simulink model "manip_levitation"  (Simulink 7.2)
settings: Solver=ode1  SolverMode=SingleTasking  StartTime=0.0  StopTime=Inf  FixedStep=1/1000  RelTol=1e-3
PostLoadFcn:
  | , if any(exist('dsrtsu_mdlpostloadfcn', 'file') == [2, 3, 6]), try dsrtsu_mdlpostloadfcn('Execute', bdroot); catch fprintf('Error in PostLoadFcn (dsrtsu_mdlpostloadfcn) for model "%s":\n %s\n', bdroot, lasterr); end, end,
libraries: rti4201serlib x3, rtilibm x1
settings Model: DSRTSU_INTERNAL_RTI_VER=330  DSRTSU_INTERNAL_RTI_TYPE=rti1005  Creator=stephane.oster  LastModifiedBy=joel.abadie  ExtModeTrigMode=oneshot  ExtModeArmWhenConnect=off  BufferReuse=off
settings OptimizationCC: BlockReduction=off  ConditionallyExecuteInputs=off  InlineInvariantSignals=on  OptimizeBlockIOStorage=off  BufferReuse=off  ExpressionFolding=off  LocalBlockOutputs=off  InitFltsAndDblsToZero=on
settings DebuggingCC: SaveWithParameterizedLinksMsg=none  SignalResolutionControl=TryResolveAllWithWarning  MultiTaskDSMMsg=warning  MultiTaskCondExecSysMsg=none  MultiTaskRateTransMsg=warning  TasksWithSamePriorityMsg=none  StrictBusMsg=None
settings HardwareCC: ProdIntDivRoundTo=Zero  ProdEndianess=BigEndian  ProdHWDeviceType=Specified  TargetIntDivRoundTo=Zero  TargetEndianess=BigEndian
settings RTWCC: SystemTargetFile=rti1005.tlc  MakeCommand=make_rti  TemplateMakefile=rti1005.tmf  Description=dSPACE DS1005 Hardware Platform  RTWVerbose=off  ProcessScript=rti1005_make_rtw_hook  CustomInclude=g:\bin_jabadie  IncludeERTFirstTime=on
settings STFCustomTargetCC: SystemTargetFile=rti1005.tlc
settings GRTTargetCC: CompOptLevelCompliant=off  MatFileLogging=off  ExtModeMexFile=noextcomm
settings CustomProperty: DataType=RTWOptions_EnumType_C__dSPACE_matlab_rti1005_tlc_rti1005_InitialSimState  Value=RUN
settings EnumStrPairs: String=RUN

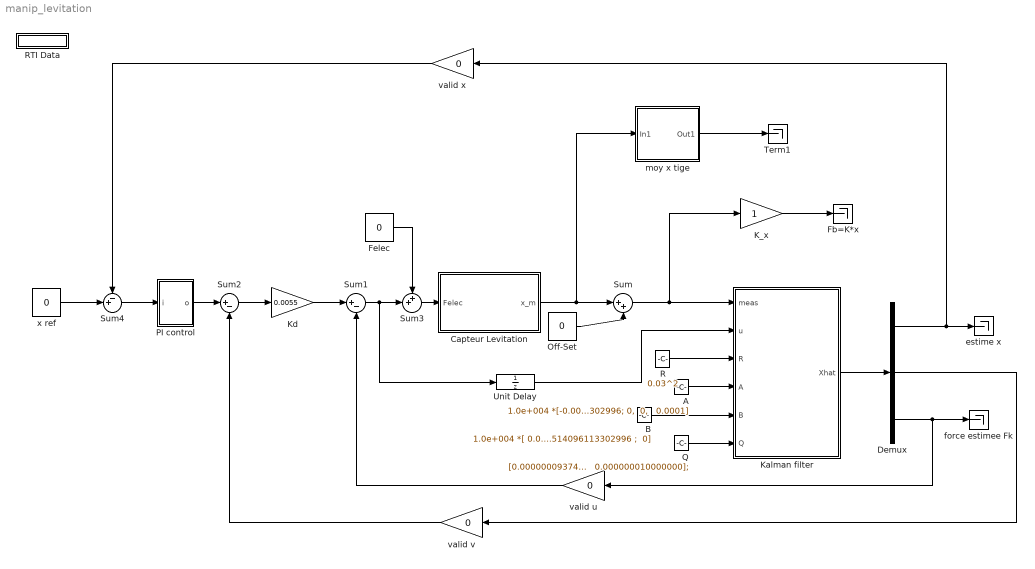
== system manip_levitation ==
  A : Constant  Value="1.0e+004 *[-0.000041693801048, 0.000000021197346, 0.000610749142449; -0.351270298286295, -0.000044721993275, 1.514096113302996; 0,  0,   0.0001]"
  B : Constant  Value=|
      | 1.0e+004 *[ 0.000610749142449;
      |    1.514096113302996;
      |  0]
  Capteur Levitation : Subsystem
  Demux : Demux  Outputs=3
  Fb=K*x : Terminator
  Felec : Constant  Value=0  OutDataType=sfix(16)  OutScaling=2^0
  K_x : Gain  ParameterDataType=sfix(16)  ParameterScaling=2^0  OutDataType=sfix(16)  OutScaling=2^0
  Kalman filter : Stateflow chart  TreatAsAtomicUnit=on
  Kd : Gain  Gain=0.0055  ParameterDataType=sfix(16)  ParameterScaling=2^0  OutDataType=sfix(16)  OutScaling=2^0
  Off-Set : Constant  Value=0  OutDataType=sfix(16)  OutScaling=2^0
  PI control : Subsystem
  Q : Constant  Value=|
      | [0.000000093740541   0.000373014515003   0.000000023776859;
      |    0.000373014515003   1.757821222396016   0.000122149828490;
      |    0.000000023776859,   0.000122149828490,   0.000000010000000];
  R : Constant  Value=0.03^2
  RTI Data : Subsystem  Tag=struct('RTIDataServer',struct('RTIModelDescription','struct(''main'',''manip_levitation'',''sub'','''',''isMp'',0)'))  LoadFcn="if exist('rtidc'), try,  rtidc('DataHostBlockClbLoad', gcbh); catch, disp(['Warning: ''LoadFcn'' for RTI Data block failed: ' lasterr]); end, end,"
      settings: CopyFcn="if exist('rtidc'), try,  rtidc('DataHostBlockClbCopy', gcbh); catch, disp(['Warning: ''CopyFcn'' for RTI Data block failed: ' lasterr]); end, end,"  DeleteFcn="if exist('rtidc'), try,  rtidc('DataHostBlockClbDelete', gcbh); catch, disp(['Warning: ''DeleteFcn'' for RTI Data block failed: ' lasterr]); end, end,"  ModelCloseFcn="if exist('rtidc'), try,  rtidc('DataHostBlockClbModelClose', gcbh); catch, disp(['Warning: ''ModelCloseFcn'' for RTI Data block failed: ' lasterr]); end, end,"  PreSaveFcn="if exist('rtidc'), try,  rtidc('DataHostBlockClbPreSave', gcbh); catch, disp(['Warning: ''PreSaveFcn'' for RTI Data block failed: ' lasterr]); end, end,"  PostSaveFcn="if exist('rtidc'), try,  rtidc('DataHostBlockClbPostSave', gcbh); catch, disp(['Warning: ''PostSaveFcn'' for RTI Data block failed: ' lasterr]); end, end,"  NameChangeFcn="if exist('rtidc'), try,  rtidc('DataHostBlockClbNameChange', gcbh); catch, disp(['Warning: ''NameChangeFcn'' for RTI Data block failed: ' lasterr]); end, end,"
      mask Type: RTI_DATA_HOST
      mask Description:
      | RTI Data Block.
      | This block is used by RTI to store internal model-dependent data.
      | Please keep this block on the root level of the model. Deleting this block will result in data loss.
      | 
      | NEVER DELETE OR COPY THIS BLOCK!
      mask Help:
      | RTI Data Block.
      | This block is used by RTI to store internal model-dependent data.
      | Please keep this block on the root level of the model. Deleting this block will result in data loss.
      | 
      | NEVER DELETE OR COPY THIS BLOCK!
      mask Display:
      | text(0.5, 0.5, 'RTI Data', 'HorizontalAlignment', 'center');
      | plot([1 0]);
  Sum : Sum  Inputs=|++  OutDataType=sfix(16)  OutScaling=2^0
  Sum1 : Sum  Inputs=|+-  OutDataType=sfix(16)  OutScaling=2^0
  Sum2 : Sum  Inputs=|+-  OutDataType=sfix(16)  OutScaling=2^0
  Sum3 : Sum  Inputs=++|  OutDataType=sfix(16)  OutScaling=2^0
  Sum4 : Sum  Inputs=-+|  OutDataType=sfix(16)  OutScaling=2^0
  Term1 : Terminator
  Unit Delay : UnitDelay  SampleTime=-1
  estime x : Terminator
  force estimee Fk : Terminator
  moy x tige : Subsystem  mask(s fonction jabadie){duree=2, T_m=0.01, to=2}
      mask prompts: duree "duree du moyennage (s)"; T_m "periode d echatillonage moyennage (s)"; to "constante de temp du filtre (s)"
      mask help:
      | sort une valeur moyenne d'un signal
      | sur une duree donnee puis applique un filtre
      | du premier ordre
  valid u : Gain  Orientation=left  Gain=0  ParameterDataType=sfix(16)  ParameterScaling=2^0  OutDataType=sfix(16)  OutScaling=2^0
  valid v : Gain  Orientation=left  Gain=0  ParameterDataType=sfix(16)  ParameterScaling=2^0  OutDataType=sfix(16)  OutScaling=2^0
  valid x : Gain  Orientation=left  Gain=0  ParameterDataType=sfix(16)  ParameterScaling=2^0  OutDataType=sfix(16)  OutScaling=2^0
  x ref : Constant  Value=0  OutDataType=sfix(16)  OutScaling=2^0
  wires:
  Demux/1 -> estime x/1, valid x/1
  Demux/3 -> force estimee Fk/1, valid u/1
  Sum/1 -> K_x/1, Kalman filter/1(meas)
  Off-Set/1 -> Sum/2
  moy x tige/1(Out1) -> Term1/1
  K_x/1 -> Fb=K*x/1
  Capteur Levitation/1(x_m) -> Sum/1, moy x tige/1(In1)
  Sum1/1 -> Unit Delay/1, Sum3/2
  Kalman filter/1(Xhat) -> Demux/1
  Demux/2 -> valid v/1
  R/1 -> Kalman filter/3(R)
  B/1 -> Kalman filter/5(B)
  A/1 -> Kalman filter/4(A)
  Q/1 -> Kalman filter/6(Q)
  Unit Delay/1 -> Kalman filter/2(u)
  Felec/1 -> Sum3/1
  Sum3/1 -> Capteur Levitation/1(Felec)
  PI control/1(o) -> Sum2/1
  Sum2/1 -> Kd/1
  Kd/1 -> Sum1/1
  valid u/1 -> Sum1/2
  Sum4/1 -> PI control/1(i)
  x ref/1 -> Sum4/2
  valid v/1 -> Sum2/2
  valid x/1 -> Sum4/1

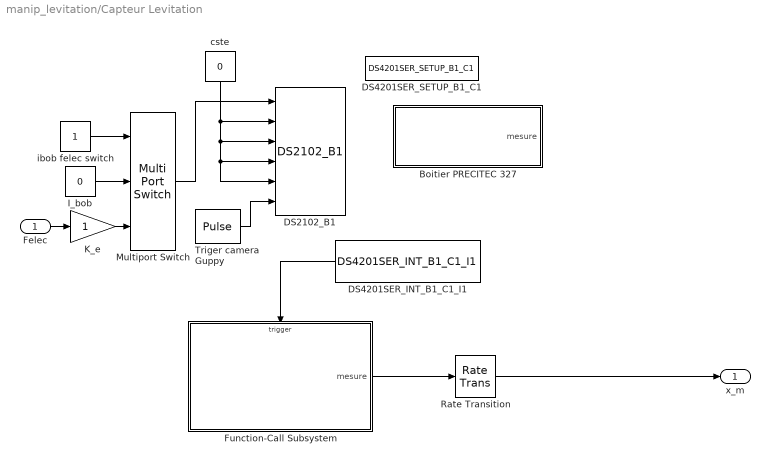
== system manip_levitation/Capteur Levitation ==
  Felec : Inport
  Boitier PRECITEC 327 : Subsystem
  DS2102_B1 : rtilibm/DS2102/DS2102_B1  SystemSampleTime=-1  BoardNo=1  Range=[10 10 10 10 10 0]  IOErrorMode=[1 1 1 1 1 1]  DeglitcherMode=[0 0 0 0 0 0]  InitValue=[0 0 0 0 0 0]  TermMode=[1 1 1 1 1 1]  TermValue=[0 0 0 0 0 0]  DialogFcn=gui2102  UnitName={'DS2102_B'}  UnitValues={ 1 }  DSProperties=struct('RTI',struct('Version',uint32(1),'BlockType',struct('isSLSource',uint8(0),'isSLSink',uint8(1),'isHWSource',uint8(0),'isHWSink',uint8(1),'isSetup',uint8(0),'isInline',uint8(1),'isNonInline',uint8(0),'isInterrupt',uint8(0),'isChannelwise',uint8(0)),'IOBoardType','DS2102','UnitType','DAC','Identifier','DAC','DialogType','ML','BlockSet','NONE','SlaveProcessor','NONE'))
  DS4201SER_INT_B1_C1_I1 : rti4201serlib/DS4201SER_INT_B1_C1_I1  Orientation=left  SystemSampleTime=-1  Reserved1=[]  Reserved2=[]  Reserved3=[]  Reserved4=[]  DSProperties=struct('RTI',struct('IOBoardType',{{'DS4201','SER'}},'SlaveProcessor','NONE','Version',uint32(3),'BlockType',struct('isSLSource',uint8(1),'isSLSink',uint8(0),'isHWSource',uint8(0),'isHWSink',uint8(0),'isSetup',uint8(0),'isInline',uint8(1),'isNonInline',uint8(0),'isInterrupt',uint8(1),'isChannelwise',uint8(1)),'UnitType','GENSER','Identifier','SERINT','DialogType','ML','BlockSet','NONE','RelationId',struct('TH',struct('BlockId','HWINT'))))  RTIBlockInterface=struct('BlockDisplay',{{['DS4201 SER Interrupt\n Board 1 Channel 1\nReceive Interrupt'],'center'}},'BlockName',struct('Token',{{'DS4201SER_INT_B','_C','_I'}},'BlockParam',{{'BoardNo','ChannelNo','IntType'}}),'OutputPortsWidth',int32(1),'OutputPortsActive',1,'OutputPortsName',{{[' ']}},'IconTransparency','off','ParameterTunableNames',{{}},'InitLevel',3,'DialogFcn','guigenserserint','MaskDescription',['To make the interrupts of the UART serial interface available as trigger source.'],'FunctionCall',uint32(0),'Options',{{'SS_OPTION_FORCE_NONINLINED_FCNCALL','SS_OPTION_ASYNCHRONOUS_INTERRUPT'}})  RTIBlockParameters=struct('Class',{{'UART','OFF',[]}},'ClassType',{{1,'OFF',[]}},'BoardType',{{'UART','OFF',[]}},'ThIntNo',{{1,'OFF',[1 4]}},'ThSubIntNo',{{0,'ON',[0 4]}},'ThSrcSgnName',{{['UART RX SW FIFO interrupt'],'OFF',[]}},'IntMode',{{0,'OFF',[]}},'TLCFileName',{{'rti_hwinterrupt','OFF',[]}},'PHSBoardBaseId',{{'DS4201S','OFF',[]}},'BoardNo',{{1,'ON',[1 16]}},'ChannelNo',{{1,'ON',[1 4]}},'ChannelNumOf',{{4,'OFF',[]}},'ThBlk',{{['struct(''blkh'',12.0009765625,''srcId'',''4201SB1I0S0'',''srcSgnId'',''4201SB1I0S0'',''intervalTmrBlockId'',[],''srcSgnName'',[''DS4201S_B1 UART RX SW FIFO interrupt''],''srcCpuId'','''',''isSrcCpu'',1,''isTargetCpu'',1,''srcOnMasterCpu'',1,''boardType'',''DS4201S'',''boardTypeNo'',''4201S'',''boardNo'',1,''intNo'',0,''subIntNo'',0,''period'',0,''entryPoint'',''rti_taskFcn001'',''blockName'',''DS4201SER_INT_B1_C1_I1'',''taskNameDisplayExt'','''',''taskType'',''HWINT'',''groupId'',''SERINT'',''hookFcn'',''NULL'',''isTimerTaskSrc'',0,''service'','''',''mpBlkId'','''',''taskPriorityPreConfig'',''none'',''taskPriority'',-1,''taskSortWeighting'',[],''taskSchedulingPolicy'',''FCFS'',''taskOvrPreConfig'',''none'',''taskOvrStrategy'',1,''taskOvrQueueSize'',1,''taskVisibility'',''on'',''taskGroupId'','''',''taskGroupDisplayOrder'',[],''serviceDynamicGen'',0,''disableCodeGen'',0)'],'OFF',[]}},'IntType',{{1,'ON',[1 4]}},'ReceiveIntLevelFifo',{{'4','OFF',[]}},'IntTypeMacro',{{'DSSER_TRIGGER_LEVEL_SUBINT_MASK','OFF',[]}},'FifoSizeDefault',{{64,'OFF',[]}})  RTISFcnParameters=struct('BoardNo','double','ChannelNo','double','ThIntNo','double','ThSubIntNo','double','ThBlk','struct','IntType','double','ReceiveIntLevelFifo','double','TLCFileName','char','IntTypeMacro','char')  RTIBlockParaDefault=struct('Class','UART','ClassType',1,'BoardType','UART','ThIntNo',1,'ThSubIntNo',0,'ThSrcSgnName',['RX SW FIFO interrupt'],'IntMode',0,'TLCFileName','rti_hwinterrupt','PHSBoardBaseId','DS4201S','BoardNo',1,'ChannelNo',1,'ChannelNumOf',4,'ThBlk',['struct(''srcSgnId'', '''')'],'IntType',1,'ReceiveIntLevelFifo',1,'IntTypeMacro','DSSER_TRIGGER_LEVEL_SUBINT_MASK','FifoSizeDefault',64)
  DS4201SER_SETUP_B1_C1 : rti4201serlib/DS4201SER_SETUP_B1_C1  SystemSampleTime=-1  Reserved1=[]  Reserved2=[]  Reserved3=[]  Reserved4=[]  DSProperties=struct('RTI',struct('Version',uint32(2),'IOBoardType',{{'DS4201','SER'}},'SlaveProcessor','NONE','BlockType',struct('isSLSource',uint8(0),'isSLSink',uint8(0),'isHWSource',uint8(0),'isHWSink',uint8(0),'isSetup',uint8(1),'isInline',uint8(1),'isNonInline',uint8(0),'isInterrupt',uint8(0),'isChannelwise',uint8(1)),'UnitType','GENSER','Identifier','SETUP','DialogType','ML','BlockSet','NONE'))  RTIBlockInterface=struct('BlockName',struct('Token',{{'DS4201SER_SETUP_B','_C'}},'BlockParam',{{'BoardNo','ChannelNo'}}),'BlockDisplay',{{['Serial Setup'],'center'}},'IconTransparency','off','ParameterTunableNames',{{}},'InitLevel',1,'DialogFcn','guigensersetup','MaskDescription',['To set the global specifications for the UART interface.'])  RTIBlockParameters=struct('ParityMode',{{1,'OFF',[1 3]}},'TransceiverMode',{{[1;1;1;1],'OFF',[]}},'QuartzFrequency',{{'1843200','OFF',[]}},'BoardNo',{{1,'ON',[1 16]}},'ChannelNo',{{1,'ON',[1 4]}},'ChannelNumOf',{{4,'OFF',[]}},'BaudRate',{{'115200','OFF',[]}},'DataBitsNumOf',{{4,'OFF',[1 4]}},'StopBitsNumOf',{{1,'OFF',[1 3]}},'ReceiveIntLevelUart',{{2,'OFF',[1 4]}},'AutoflowMode',{{0,'OFF',[]}},'FifoSize',{{'256','OFF',[]}},'ReceiveIntLevelFifo',{{0,'OFF',[]}},'FifoOverrunMode',{{2,'OFF',[]}},'FifoBlockSize',{{'4','OFF',[]}},'TermMode',{{1,'OFF',[]}},'TLCFileName',{{'rtigensersetup','OFF',[]}})  RTISFcnParameters=struct('BoardNo','double','ChannelNo','double','ChannelNumOf','double','BaudRate','double','DataBitsNumOf','double','StopBitsNumOf','double','ParityMode','double','TransceiverMode','double','ReceiveIntLevelUart','double','AutoflowMode','double','FifoSize','double','ReceiveIntLevelFifo','double','FifoBlockSize','double','TermMode','double','QuartzFrequency','double','TLCFileName','char')  RTIBlockParaDefault=struct('ParityMode',1,'TransceiverMode',[1;1;1;1],'QuartzFrequency',1843200,'BoardNo',1,'ChannelNo',1,'ChannelNumOf',4,'BaudRate',115200,'DataBitsNumOf',4,'StopBitsNumOf',1,'ReceiveIntLevelUart',4,'AutoflowMode',0,'FifoSize',64,'ReceiveIntLevelFifo',0,'FifoOverrunMode',1,'FifoBlockSize',0,'TermMode',1,'TLCFileName','rtigensersetup')
  Function-Call Subsystem : Subsystem  TreatAsAtomicUnit=on
  I_bob : Constant  Value=0  OutDataType=sfix(16)  OutScaling=2^0
  K_e : Gain  ParameterDataType=sfix(16)  ParameterScaling=2^0  OutDataType=sfix(16)  OutScaling=2^0
  Multiport Switch : MultiPortSwitch  Inputs=2  OutDataType=sfix(16)  OutScaling=2^0
  Rate Transition : RateTransition  Deterministic=off  OutPortSampleTimeOpt=Inherit
  Triger camera Guppy : DiscretePulseGenerator  PulseType=Time based  Amplitude=0.5  Period=1  PulseWidth=50
  cste : Constant  Orientation=down  Value=0  OutDataType=sfix(16)  OutScaling=2^0
  ibob felec switch : Constant  OutDataType=sfix(16)  OutScaling=2^0
  x_m : Outport
  wires:
  cste/1 -> DS2102_B1/2, DS2102_B1/3, DS2102_B1/4, DS2102_B1/5
  Felec/1 -> K_e/1
  ibob felec switch/1 -> Multiport Switch/1
  K_e/1 -> Multiport Switch/3
  I_bob/1 -> Multiport Switch/2
  DS4201SER_INT_B1_C1_I1/1 -> Function-Call Subsystem/Trigger
  Function-Call Subsystem/1(mesure) -> Rate Transition/1
  Rate Transition/1 -> x_m/1
  Multiport Switch/1 -> DS2102_B1/1
  Triger camera Guppy/1 -> DS2102_B1/6

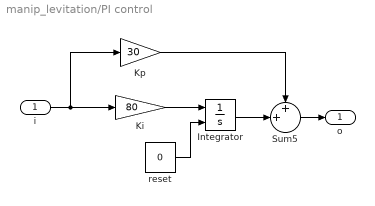
== system manip_levitation/PI control ==
  i : Inport
  Integrator : Integrator  ExternalReset=level
  Ki : Gain  Gain=80  ParameterDataType=sfix(16)  ParameterScaling=2^0  OutDataType=sfix(16)  OutScaling=2^0  SaturateOnIntegerOverflow=on  OutDataTypeStr=Inherit: Same as input  ParamDataTypeStr=Inherit: Same as input
  Kp : Gain  Gain=30  ParameterDataType=sfix(16)  ParameterScaling=2^0  OutDataType=sfix(16)  OutScaling=2^0  SaturateOnIntegerOverflow=on  OutDataTypeStr=Inherit: Same as input  ParamDataTypeStr=Inherit: Same as input
  Sum5 : Sum  Inputs=++|  OutDataType=sfix(16)  OutScaling=2^0  SaturateOnIntegerOverflow=on  InputSameDT=on  OutDataTypeStr=Inherit: Same as first input
  reset : Constant  Value=0  OutDataType=sfix(16)  OutScaling=2^0
  o : Outport
  wires:
  Ki/1 -> Integrator/1
  Kp/1 -> Sum5/1
  Integrator/1 -> Sum5/2
  i/1 -> Ki/1, Kp/1
  Sum5/1 -> o/1
  reset/1 -> Integrator/2

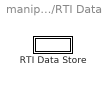
== system manip_levitation/RTI Data ==
  RTI Data Store : Subsystem  Tag="struct('public',struct('sub',struct('name',{{'manip_levitation'}},'data',{{struct('TH',struct('thTaskInfo',struct('taskType',{'TIMER','HWINT','TMRINT','SWINT'},'tasksNumOf',{1,1,0,0},'srcIds',{{'TIMERA'},{'4201SB1I0S0'},{},{}},'entryPoints',{{'rti_TIMERA'},{'rti_taskFcn001'},{},{}},'taskNames',{{['Timer Task 1']},{'DS4201SER_INT_B1_C1_I1'},{},{}})),'th_tc',struct('dataType',{'TASK','TASK'},'taskGroupId',{'',''},'taskGroupList',{{},{}},'taskSchedulingPolicy',{'FCFS','FCFS'},'taskType',{'TIMER','HWINT'},'blkh',{-1,['manip_levitation/Capteur Levitation/DS4201SER_INT_B1_C1_I1']},'srcId',{'TIMERA','4201SB1I0S0'},'srcSgnName',{['Timer A interrupt'],['DS4201S_B1 UART RX SW FIFO interrupt']},'srcCpuName',{'',''},'taskName',{['Timer Task 1  [0.001] s'],'DS4201SER_INT_B1_C1_I1'},'taskNameDisplayExt',{'',''},'smplTime',{0.001,0},'smplTimeOffs',{0,0},'hasFixedPriority',{0,0},'priority',{1,2},'hasFixedOvc',{0,0},'ovcType',{1,1},'ovcMax',{0,1}),'tc_th',struct('dataType',{'TASK','TASK'},'taskGroupId',{'',''},'taskGroupList',{{},{}},'taskSchedulingPolicy',{'FCFS','FCFS'},'taskType',{'TIMER','HWINT'},'blkh',{-1,['manip_levitation/Capteur Levitation/DS4201SER_INT_B1_C1_I1']},'srcId',{'TIMERA','4201SB1I0S0'},'srcSgnName',{['Timer A interrupt'],['DS4201S_B1 UART RX SW FIFO interrupt']},'srcCpuName',{'',''},'taskName',{['Timer Task 1  [0.001] s'],'DS4201SER_INT_B1_C1_I1'},'taskNameDisplayExt',{'',''},'smplTime',{0.001,0},'smplTimeOffs',{0,0},'hasFixedPriority',{0,0},'priority',{1,2},'hasFixedOvc',{0,0},'ovcType',{1,1},'ovcMax',{0,1}))}})),'private',struct('version',struct('dsVer',uint32(2)),'access',struct('modified',['21-May-2019 12:33:58'],'type','Model','isPerm',1)))"
      mask Type: RTI_DATA_STORE
      mask Description:
      | RTI Data Store Block. This block is used by RTI to store internal model dependent data. Deleting this block will result in data loss.
      | 
      | NEVER DELETE, COPY, OR MODIFY THIS BLOCK!
      mask Help:
      | RTI Data Store Block. This block is used by RTI to store internal model dependent data. Deleting this block will result in data loss.
      | 
      | NEVER DELETE, COPY, OR MODIFY THIS BLOCK!
      mask Display: text(0.5, 0.5, ' ', 'HorizontalAlignment', 'center');

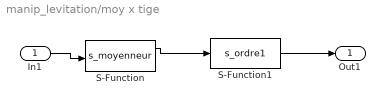
== system manip_levitation/moy x tige ==
  In1 : Inport
  S-Function : S-Function  FunctionName=s_moyenneur  Parameters=duree,T_m  EnableBusSupport=off
  S-Function1 : S-Function  FunctionName=s_ordre1  Parameters=1,to,0  EnableBusSupport=off
  Out1 : Outport
  wires:
  In1/1 -> S-Function/1
  S-Function/1 -> S-Function1/1
  S-Function1/1 -> Out1/1

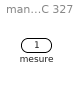
== system manip_levitation/Capteur Levitation/Boitier PRECITEC 327 ==
  mesure : Outport
  wires:
  ? -> mesure/1

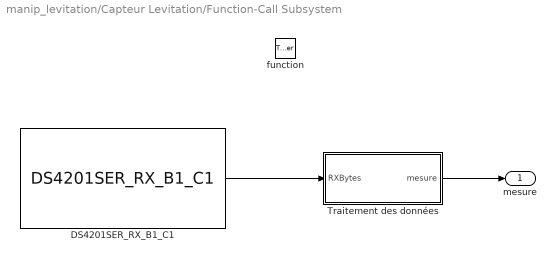
== system manip_levitation/Capteur Levitation/Function-Call Subsystem ==
  function : TriggerPort  TriggerType=function-call
  DS4201SER_RX_B1_C1 : rti4201serlib/DS4201SER_RX_B1_C1  SystemSampleTime=-1  Reserved1=[]  Reserved2=[]  Reserved3=[]  Reserved4=[]  DSProperties=struct('RTI',struct('IOBoardType',{{'DS4201','SER'}},'SlaveProcessor','NONE','Version',uint32(1),'BlockType',struct('isSLSource',uint8(1),'isSLSink',uint8(1),'isHWSource',uint8(0),'isHWSink',uint8(1),'isSetup',uint8(0),'isInline',uint8(1),'isNonInline',uint8(0),'isInterrupt',uint8(0),'isChannelwise',uint8(1)),'UnitType','GENSER','Identifier','RECEIVE','DialogType','ML','BlockSet','NONE'))  RTIBlockInterface=struct('BlockName',struct('Token',{{'DS4201SER_RX_B','_C'}},'BlockParam',{{'BoardNo','ChannelNo'}}),'InputPortsWidth',int32(1),'InputPortsActive',0,'InputPortsDataType',{{'SS_UINT32'}},'InputPortsName',{{'NumBytes'}},'OutputPortsWidth',int32([4 1 1]),'OutputPortsActive',[1 0 0],'OutputPortsDataType',{{'SS_UINT8','SS_UINT32','SS_INT32'}},'OutputPortsName',{{'RXBytes','NumRXBytes','Status'}},'BlockDisplay',{{['Serial Receive'],'center'}},'IconTransparency','on','ParameterTunableNames',{{}},'InitLevel',2,'DialogFcn','guigenserreceive','MaskDescription',['To read data from the UART SW FIFO.'])  RTIBlockParameters=struct('BoardNo',{{1,'ON',[1 16]}},'ChannelNo',{{1,'ON',[1 4]}},'ChannelNumOf',{{4,'OFF',[]}},'ReceptionDataMode',{{2,'OFF',[]}},'ParamTunableMode',{{2,'OFF',[]}},'BytesRefNumOfT',{{'6','OFF',[1 inf]}},'BytesRefNumOfNT',{{'4','OFF',[1 inf]}},'BytesRefNumOfMax',{{'6','OFF',[1 inf]}},'BytesRefNumOfMode',{{1,'OFF',[]}},'BytesActNumOfMode',{{0,'OFF',[]}},'ReceptionStatusMode',{{0,'OFF',[]}},'FifoSizeDefault',{{64,'OFF',[]}},'TLCFileName',{{'rtigenserreceive','OFF',[]}})  RTISFcnParameters=struct('BoardNo','double','ChannelNo','double','ChannelNumOf','double','ReceptionDataMode','double','ParamTunableMode','double','BytesRefNumOfT','double','BytesRefNumOfNT','double','BytesRefNumOfMax','double','BytesRefNumOfMode','double','BytesActNumOfMode','double','ReceptionStatusMode','double','TLCFileName','char')  RTIBlockParaDefault=struct('BoardNo',1,'ChannelNo',1,'ChannelNumOf',4,'ReceptionDataMode',1,'ParamTunableMode',1,'BytesRefNumOfT',1,'BytesRefNumOfNT',1,'BytesRefNumOfMax',1,'BytesRefNumOfMode',0,'BytesActNumOfMode',1,'ReceptionStatusMode',1,'FifoSizeDefault',64,'TLCFileName','rtigenserreceive')
  Traitement des données : Stateflow chart
  mesure : Outport  OutDataType=sfix(16)  OutScaling=2^0
  wires:
  DS4201SER_RX_B1_C1/1 -> Traitement des données/1(RXBytes)
  Traitement des données/1(mesure) -> mesure/1

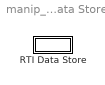
== system manip_levitation/RTI Data/RTI Data Store ==
  RTI Data Store : Subsystem
      mask Type: RTI_DATA_STORE
      mask Description:
      | RTI Data Store Block. This block is used by RTI to store internal model dependent data. Deleting this block will result in data loss.
      | 
      | NEVER DELETE, COPY, OR MODIFY THIS BLOCK!
      mask Help:
      | RTI Data Store Block. This block is used by RTI to store internal model dependent data. Deleting this block will result in data loss.
      | 
      | NEVER DELETE, COPY, OR MODIFY THIS BLOCK!
      mask Display: text(0.5, 0.5, ' ', 'HorizontalAlignment', 'center');

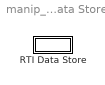
== system manip_levitation/RTI Data/RTI Data Store/RTI Data Store ==
  RTI Data Store : Subsystem
      mask Type: RTI_DATA_STORE
      mask Description:
      | RTI Data Store Block. This block is used by RTI to store internal model dependent data. Deleting this block will result in data loss.
      | 
      | NEVER DELETE, COPY, OR MODIFY THIS BLOCK!
      mask Help:
      | RTI Data Store Block. This block is used by RTI to store internal model dependent data. Deleting this block will result in data loss.
      | 
      | NEVER DELETE, COPY, OR MODIFY THIS BLOCK!
      mask Display: text(0.5, 0.5, ' ', 'HorizontalAlignment', 'center');

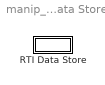
== system manip_levitation/RTI Data/RTI Data Store/RTI Data Store/RTI Data Store ==
  RTI Data Store : Subsystem
      mask Type: RTI_DATA_STORE
      mask Description:
      | RTI Data Store Block. This block is used by RTI to store internal model dependent data. Deleting this block will result in data loss.
      | 
      | NEVER DELETE, COPY, OR MODIFY THIS BLOCK!
      mask Help:
      | RTI Data Store Block. This block is used by RTI to store internal model dependent data. Deleting this block will result in data loss.
      | 
      | NEVER DELETE, COPY, OR MODIFY THIS BLOCK!
      mask Display: text(0.5, 0.5, ' ', 'HorizontalAlignment', 'center');

== system manip_levitation/RTI Data/RTI Data Store/RTI Data Store/RTI Data Store/RTI Data Store ==

== matlab function Capteur Levitation/Function-Call Subsystem/Traitement des données ==
  data: RXBytes input double; mesure output double
function mesure = fcn(RXBytes)

% V0 ecrite par JAbadie le 5/12/2014 
% rappel config DS4201SER SETUP bloc
% onglet UART : RS232 115200 Baud, Data Bits 8, Stop bits 1, Parity No,
% Copy data to RX SW FIFO after reception of 4 bytes at least
% onglet FIFO : Replace old data with FIFO method, bloc size 4 bytes

% rappel config DS4201SER_RX bloc
% Reception mode : skip read operation
% Parameter flexibility : non tunable
% Number of bytes 4

% Penser a charger la config MANIP PIEZO sur le boitier precitec
% CONFIG -> Service functions > Load setup

% Remarque en cas de mauvaise synchro au demarage de la liaison
% la mesure reste a zero c'est voulu.
% redémarer à nouveau !

% Le test de la laison s'effectue avec le bloc Precitec du modele
% G:\Manip_piezo\test_connect_precitec.mdl
% G:\Manip_piezo\visuliaisonprecitec.lay

code=double(RXBytes)

if code(1)==255 && code(2)==255
    MSB = code(3);
    LSB = code(4);
elseif code(3)==255 && code(4)==255
    MSB = code(1);
    LSB = code(2);  
elseif code(1)==255 && code(4)==255
    MSB = code(2);
    LSB = code(3);
else
    MSB = 0;
    LSB = 0;
end

mesure  = ((MSB + LSB/255)*300)/128*1e-6;

== matlab function Kalman filter ==
  data: meas input double; u input double; R input double; Xhat output double; A input double; B input double; Q input double
function Xhat = kalman(meas,u,R,A,B,Q)

% In this Kalman Filter we followed a Prediction-Estimation scheme

% Initialization
persistent P;
persistent xest;

%initialisations
if isempty(P)
    xest = [0; 0; 0];  %on suppose la tige au repos et la force nulle
    P = [ 2 0 0; 0 10 0; 0 0 50];% Matrice de covariance initiale estimï¿½e de l'ï¿½tat x[0] de la tige et de la force:
end

C=[1 0 0];

% Etape de prediction (nota : pas de "commande")
xpre = A*xest + B*u;
Ppre = A*P*A' + Q;

% calcul du gain de Kalman (non stationnaire)
K = (Ppre*C')*inv(C*Ppre*C' + R);

% Etape d'estimation a l'aide de l'observation du deplacement bruite de la tige
xest = xpre + K*(meas - C*xpre); 
P = Ppre - K*C*Ppre;
%------------------------------------------------

Xhat = xest;
%Yhatout = [meas; u; 0];
end
